simulink model "linear_arm_model"  (R2021b)
settings: Solver=VariableStepAuto  StartTime=0.0  StopTime=8  RelTol=1e-3
values from neighbouring files (symbols this model uses):
  AmpDen = [1 655.7 5.52e6]    [draft_model_variables.m]    (also in linear_model_variables.m)
  AmpNum = [2.149e7]    [draft_model_variables.m]    (also in linear_model_variables.m)
  B = 7e-4    (= 0.0007)    [draft_model_variables.m]    (also in linear_model_variables.m)
  CF = 1000    [derivative_filter.m]    (also in draft_model_variables.m = 1163; linear_model_variables.m)
  gear_i = 100    [draft_model_variables.m]    (also in linear_model_variables.m)
  J1 = 2.60    (= 2.6)    [linear_model_variables.m]
  J2 = 0.50    (= 0.5)    [linear_model_variables.m]
  K1 = 0.589    [draft_model_variables.m]    (also in linear_model_variables.m = 39.8)
  K2 = 0.0753    [draft_model_variables.m]    (also in linear_model_variables.m = 1.25)
  ka = km    (= 0.0228)    [draft_model_variables.m]    (also in linear_model_variables.m = 0.0164)
  Kd1 = 109.6356    [draft_model_variables.m]    (also in linear_model_variables.m = 0.016163066074)
  Kd2 = 99.9905    [draft_model_variables.m]    (also in linear_model_variables.m = 0.00914883559048)
  Ki1 = 1    [draft_model_variables.m]    (also in linear_model_variables.m)
  Ki2 = 1    [draft_model_variables.m]    (also in linear_model_variables.m)
  km = 22.8*1e-3    (= 0.0228)    [draft_model_variables.m]    (also in linear_model_variables.m = 0.0164)
  Kp1 = 20.9419    [draft_model_variables.m]    (also in linear_model_variables.m = 0.254768095317)
  Kp2 = 19.9995    [draft_model_variables.m]    (also in linear_model_variables.m = 0.192126266518)
  L = 0.475*1e-3    (= 0.000475)    [draft_model_variables.m]    (also in linear_model_variables.m = 0.000245)
  N = 10    [derivative_filter.m]    (also in draft_model_variables.m = 100; linear_model_variables.m = 100)
  R = 0.713    [draft_model_variables.m]    (also in linear_model_variables.m = 0.115)
  s = tf('s')    [draft_model_variables.m]    (also in linear_model_variables.m)
libraries: cstblocks x2, simulink x2
settings Model: Creator=ncamp  LastModifiedBy=ncamp

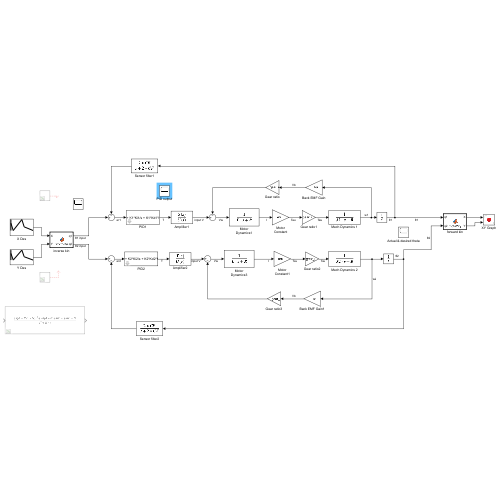
[thumbnail: Simulink's stored preview of the top-level diagram]
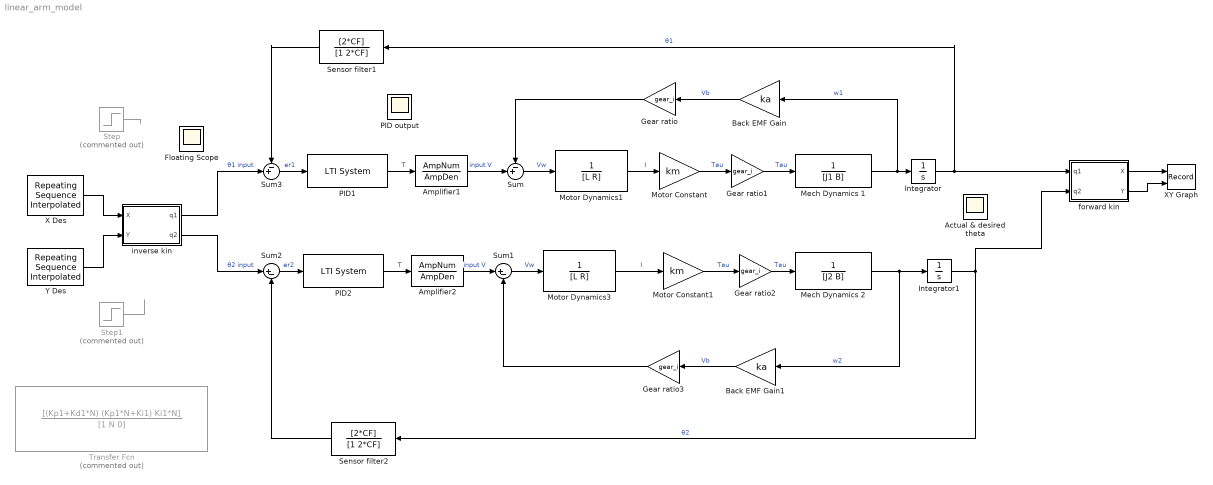
== system linear_arm_model ==
  Actual & desired theta : Scope
      settings: Floating=on
  Amplifier1 : TransferFcn  Numerator=AmpNum  Denominator=AmpDen
  Amplifier2 : TransferFcn  Numerator=AmpNum  Denominator=AmpDen
  Back EMF Gain : Gain  Gain=ka
  Back EMF Gain1 : Gain  Gain=ka
  Floating Scope : Scope
      settings: Floating=on
  Gear ratio{,1..3} (4 alike) : Gain  Gain=gear_i
  Integrator : Integrator
  Integrator1 : Integrator
  Mech Dynamics 1 : TransferFcn  Denominator=[J1 B]
  Mech Dynamics 2 : TransferFcn  Denominator=[J2 B]
  Motor Constant : Gain  Gain=km
  Motor Constant1 : Gain  Gain=km
  Motor Dynamics1 : TransferFcn  Denominator=[L R]
  Motor Dynamics3 : TransferFcn  Denominator=[L R]
  PID output : Scope
      settings: Floating=on
  PID1 : cstblocks/LTI System  sys=tf(K1*Kp1 + K1*Ki1/s + K1*Kd1*N*s/(s+N))  IC=[]
  PID2 : cstblocks/LTI System  sys=tf(K2*Kp2 + K2*Ki2/s + K2*Kd2*N*s/(s+N))  IC=[]
  Sensor filter1 : TransferFcn  Numerator=[2*CF]  Denominator=[1 2*CF]
  Sensor filter2 : TransferFcn  Numerator=[2*CF]  Denominator=[1 2*CF]
  Step : Step  Commented=on  Before=550  After=300  SampleTime=0.0001
  Step1 : Step  Commented=on  After=300  SampleTime=0.001
  Sum : Sum  Inputs=-+|
  Sum1 : Sum  Inputs=|+-
  Sum2 : Sum  Inputs=|+-
  Sum3 : Sum  Inputs=-+|
  Transfer Fcn : TransferFcn  Commented=on  Numerator=[(Kp1+Kd1*N) (Kp1*N+Ki1) Ki1*N]  Denominator=[1 N 0]
  X Des : simulink/Sources/Repeating Sequence Interpolated  OutValues=X  TimeValues=time  LookUpMeth=Interpolation-Use End Values  tsamp=0.001  OutMin=[]  OutMax=[]  OutDataTypeStr=double  OutputDataTypeScalingMode=double  OutDataType=fixdt(0,8)  OutScaling=2^-10
  XY Graph : Record  FileSettingsInternal="{\"entries\":[{\"content\":{\"excelSettings\":{\"content\":{},\"type\":\"Streamout.ExcelSettings\"}},\"type\":\"Streamout.FileSettingStorage\",\"uuid\":\"6a9b1b81-b615-47ff-9e78-6503a574d015\"}],\"packageUris\":[\"http://schema.mathworks.com/mf0/streamout_blocks/R2020a\"],\"version\":\"1.0\"}"  Layout=[1 2]  SignalsInternal="{\"entries\":[{\"content\":{\"signals\":[{\"content\":{\"blockPath\":[\"linear_arm_model/XY Graph\"],\"channel\":[],\"dimensions\":[1],\"domain\":\"linear_arm_model/XY Graph\",\"lineColor\":\"#a2142f\",\"plots\":[1],\"port\":1,\"sid\":[\"\"],\"signalID\":63,\"signalName\":\"forward kin:1\"},\"type\":\"RecordBlkView.Signal\",\"uuid\":\"2d032cc6-dc58-4401-a74f-90bd6e4e612e\"},{\"content\":{\"blockPath\":[\"linear_arm_model/XY Graph\"],\"channel\":[],\"dimensions\":[1],\"domain\":\"linear_arm_model/XY Graph\",\"lineColor\":\"#139fff\",\"plots\":[1],\"port\":2,\"sid\":[\"\"],\"signalID\":67,\"signalName\":\"forward kin:2\"},\"type\":\"RecordBlkView.Signal\",\"uuid\":\"29bd27e6-4a81-4743-8384-20c9bd1847e2\"}]},\"type\":\"RecordBlkView.InputSignals\",\"uuid\":\"0857c9eb-267e-49c3-adc7-e6c998aeaa3e\"}],\"packageUris\":[\"http://schema.mathworks.com/mf0/streamout_blocks/R2020a\"],\"version\":\"1.0\"}"  VisualizationBindings="{\"xyplotplugin\":{\"info\":[{\"series\":[{\"bindingParametersList\":[{\"parameter\":\"X-Axis\",\"signalID\":63,\"signalName\":\"forward kin:1\"},{\"parameter\":\"Y-Axis\",\"signalID\":67,\"signalName\":\"forward kin:2\"}],\"seriesID\":19959}],\"subplotID\":1}]}}"  CompatibilityTag=XY
  Y Des : simulink/Sources/Repeating Sequence Interpolated  OutValues=Y  TimeValues=time  LookUpMeth=Interpolation-Use End Values  tsamp=0.001  OutMin=[]  OutMax=[]  OutDataTypeStr=double  OutputDataTypeScalingMode=double  OutDataType=fixdt(0,8)  OutScaling=2^-10
  forward kin : MATLAB Function  TreatAsAtomicUnit=on
  inverse kin : MATLAB Function  TreatAsAtomicUnit=on
  wires:
  Back EMF Gain/1 -> Gear ratio/1  "Vb"
  Motor Dynamics1/1 -> Motor Constant/1  "I"
  Sum/1 -> Motor Dynamics1/1  "Vw"
  Back EMF Gain1/1 -> Gear ratio3/1  "Vb"
  Motor Dynamics3/1 -> Motor Constant1/1  "I"
  Sum1/1 -> Motor Dynamics3/1  "Vw"
  Sum2/1 -> PID2/1  "er2"
  PID2/1 -> Amplifier2/1  "T"
  Amplifier2/1 -> Sum1/1  "input V"
  PID1/1 -> Amplifier1/1  "T"
  Amplifier1/1 -> Sum/2  "input V"
  Sum3/1 -> PID1/1  "er1"
  Motor Constant1/1 -> Gear ratio2/1  "Tau"
  Gear ratio2/1 -> Mech Dynamics 2/1  "Tau"
  Motor Constant/1 -> Gear ratio1/1  "Tau"
  Gear ratio1/1 -> Mech Dynamics 1/1  "Tau"
  Gear ratio3/1 -> Sum1/2
  Gear ratio/1 -> Sum/1
  Mech Dynamics 1/1 -> Integrator/1, Back EMF Gain/1  "w1"
  Mech Dynamics 2/1 -> Integrator1/1, Back EMF Gain1/1  "w2"
  X Des/1 -> inverse kin/1(X)
  Y Des/1 -> inverse kin/2(Y)
  inverse kin/1(q1) -> Sum3/2  "θ1 input"
  inverse kin/2(q2) -> Sum2/1  "θ2 input"
  Integrator1/1 -> Sensor filter2/1, forward kin/2(q2)  "θ2"
  Integrator/1 -> forward kin/1(q1), Sensor filter1/1  "θ1"
  forward kin/1(X) -> XY Graph/1
  forward kin/2(Y) -> XY Graph/2
  Sensor filter2/1 -> Sum2/2
  Sensor filter1/1 -> Sum3/1
  Step/1 -> ?
  Step1/1 -> ?

== matlab function linear_arm_model/inverse kin ==
  data: X input; q1 output; Y input; q2 output
function [q1,q2] = xy2theta(X,Y)

% Inputs X,Y should be in mm
% Outputs q1, q2 are in rads

L1 = 275;   % Arm 1 length (mm)
L2 = 275;   % Arm 2 length (mm)

% Elbow down position
q1 = 2*atan((2*L1*Y - (- L1^4 + 2*L1^2*L2^2 + 2*L1^2*X^2 + 2*L1^2*Y^2 - L2^4 + 2*L2^2*X^2 + 2*L2^2*Y^2 - X^4 - 2*X^2*Y^2 - Y^4)^(1/2))/(L1^2 + 2*L1*X - L2^2 + X^2 + Y^2));
q2 =  2*atan(((- L1^2 + 2*L1*L2 - L2^2 + X^2 + Y^2)*(L1^2 + 2*L1*L2 + L2^2 - X^2 - Y^2))^(1/2)/(- L1^2 + 2*L1*L2 - L2^2 + X^2 + Y^2));


end

== matlab function linear_arm_model/forward kin ==
  data: q1 input; X output; q2 input; Y output
function [X,Y] = theta2xy(q1,q2)

L1 = 275;
L2 = 275;

X = L1*cos(q1) + L2*cos(q1 + q2);
Y = L1*sin(q1) + L2*sin(q1 + q2);

end
